simulink model "fahrenheitTo_celsiue"  (R2024b)
settings: Solver=VariableStepAuto  StartTime=0.0  StopTime=inf  RelTol=1e-3
settings Model: Creator=admin  LastModifiedBy=admin

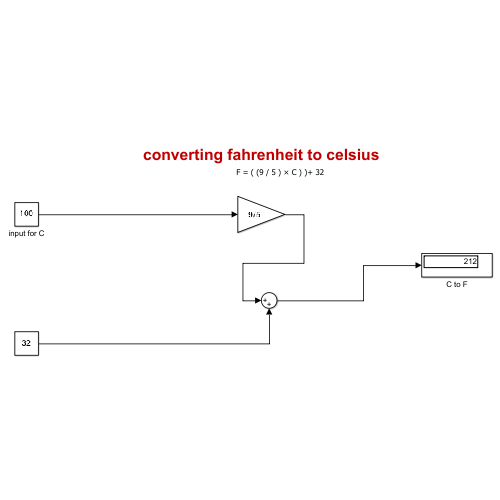
[thumbnail: Simulink's stored preview of the top-level diagram]
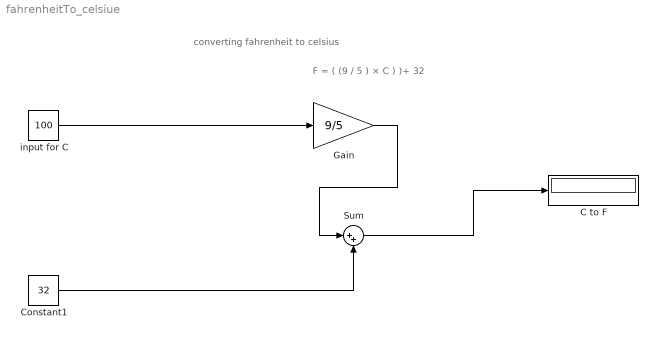
== system fahrenheitTo_celsiue ==
  note: F = ( (9 / 5 )​ × C ) )+ 32
  note: converting fahrenheit to celsius
  C to F : Display
  Constant1 : Constant  Value=32
  Gain : Gain  Gain=9/5
  Sum : Sum  Inputs=|++
  input for C : Constant  Value=100
  wires:
  input for C/1 -> Gain/1
  Gain/1 -> Sum/1
  Constant1/1 -> Sum/2
  Sum/1 -> C to F/1
